simulink model "sampleModel259"  (R2021b)
settings: Solver=VariableStepAuto  StartTime=0.0  StopTime=10.0  RelTol=1e-3
undefined symbols (not defined in the file or in its folder): DiscIntNeverNeededParam
libraries: simulink x9, slpidlib x1
settings Model: Creator=user  LastModifiedBy=user

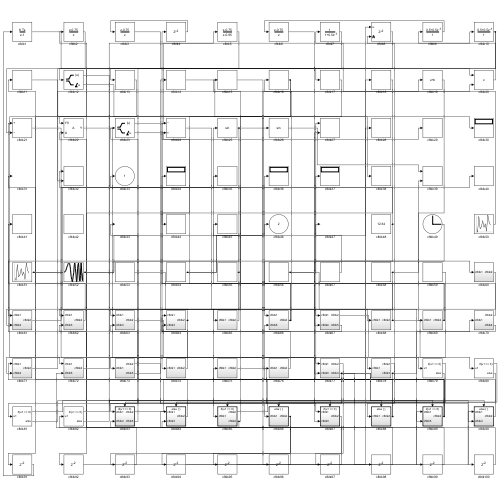
[thumbnail: Simulink's stored preview of the top-level diagram]
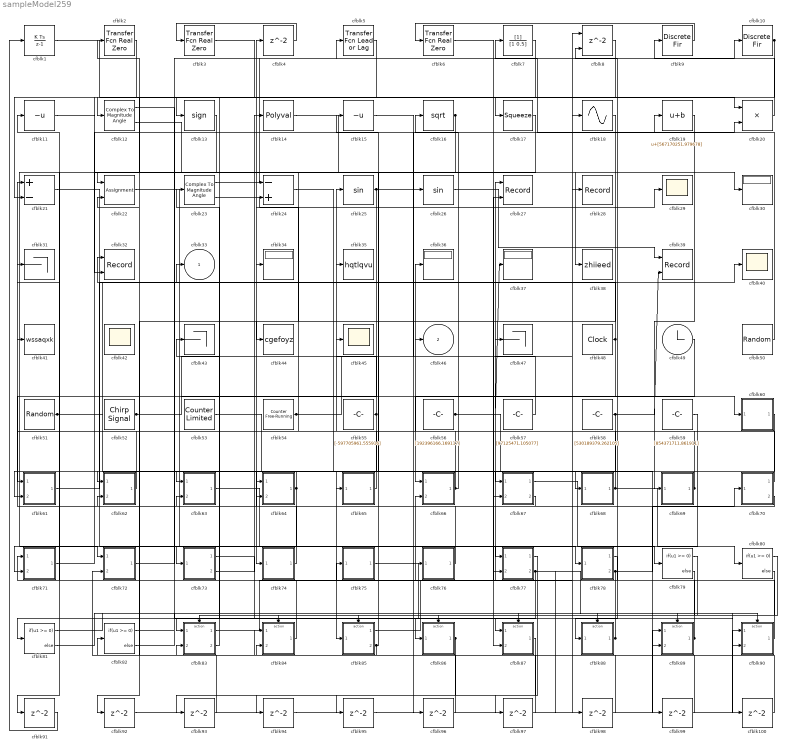
== system sampleModel259 ==
  cfblk1 : DiscreteIntegrator  ICPrevOutput=DiscIntNeverNeededParam  ICPrevScaledInput=DiscIntNeverNeededParam
  cfblk10 : DiscreteFir  SampleTime=1
  cfblk{4,91..100} (11 alike) : Delay  SampleTime=1
  cfblk11 : UnaryMinus
  cfblk12 : ComplexToMagnitudeAngle
  cfblk13 : Signum
  cfblk14 : Polyval  Coefs=[ +2.081618890e-019, -1.441693666e-014, +4.719686976e-010, -8.536869453e-006, +1.621573104e-001, -8.087801117e+001 ]
  cfblk15 : UnaryMinus
  cfblk16 : Sqrt  SaturateOnIntegerOverflow=on
  cfblk17 : Squeeze
  cfblk18 : Sin  TimeSource=Use external signal  SampleTime=0
  cfblk19 : Bias  Bias=[567170251.979678]
  cfblk2 : simulink/Discrete/Transfer Fcn Real Zero  ZeroZ=0.75  ICPrevInput=0.0  DoSatur=off
      settings: SourceProductBaseCode=SL
  cfblk20 : Product  Inputs=**
  cfblk21 : Sum  Inputs=+-
  cfblk22 : Assignment  DiagnosticForDimensions=Warning  IndexOptions=Index vector (dialog)  Indices=1  OutputSizes=1
  cfblk23 : ComplexToMagnitudeAngle
  cfblk24 : Sum  Inputs=-+
  cfblk25 : Trigonometry
  cfblk26 : Trigonometry
  cfblk27 : Record  FileSettingsInternal="{\"entries\":[{\"content\":{\"excelSettings\":{\"content\":{},\"type\":\"Streamout.ExcelSettings\"}},\"type\":\"Streamout.FileSettingStorage\",\"uuid\":\"a15bf5db-3741-4cf3-90f6-61c3119d6459\"}],\"packageUris\":[\"http://schema.mathworks.com/mf0/streamout_blocks/R2020a\"],\"version\":\"1.0\"}"  Layout=[1 1]  SignalsInternal="{\"entries\":[{\"content\":{\"signals\":[{\"content\":{\"blockPath\":[\"sampleModel259/cfblk27\"],\"channel\":[],\"dimensions\":[1],\"domain\":\"sampleModel259/cfblk27\",\"lineColor\":\"#a2142f\",\"plots\":[1],\"port\":1,\"sid\":[\"\"],\"signalID\":10726,\"signalName\":\"cfblk88\"},\"type\":\"RecordBlkView.Signal\",\"uuid\":\"dc7c6215-aa68-4dff-98e1-634e55d8342f\"},{\"content\":{\"blockPath\":[\"sampleModel259/cfblk27\"],\"channel\":[],\"dimensions\":[1],\"domain\":\"sampleModel259/cfblk27\",\"lineColor\":\"#139fff\",\"plots\":[1],\"port\":2,\"sid\":[\"\"],\"signalID\":10730,\"signalName\":\"cfblk85:1\"},\"type\":\"RecordBlkView.Signal\",\"uuid\":\"56125518-63ef-40df-9fd8-c2bea6029bef\"}]},\"type\":\"RecordBlkView.InputSignals\",\"uuid\":\"c2e7fa76-5202-4da8-ac4b-8a415a1de49b\"}],\"packageUris\":[\"http://schema.mathworks.com/mf0/streamout_blocks/R2020a\"],\"version\":\"1.0\"}"  VisualizationBindings="{\"xyplotplugin\":{\"info\":[{\"series\":[{\"bindingParametersList\":[{\"parameter\":\"X-Axis\",\"signalID\":10726,\"signalName\":\"cfblk88\"},{\"parameter\":\"Y-Axis\",\"signalID\":10730,\"signalName\":\"cfblk85:1\"}],\"seriesID\":54620}],\"subplotID\":1}]}}"  CompatibilityTag=XY
  cfblk28 : Record  FileSettingsInternal="{\"entries\":[{\"content\":{\"excelSettings\":{\"content\":{},\"type\":\"Streamout.ExcelSettings\"}},\"type\":\"Streamout.FileSettingStorage\",\"uuid\":\"feed3611-4c3d-457a-aeeb-df4a7c1a2444\"}],\"packageUris\":[\"http://schema.mathworks.com/mf0/streamout_blocks/R2020a\"],\"version\":\"1.0\"}"  SignalsInternal="{\"entries\":[{\"content\":{\"signals\":[{\"content\":{\"blockPath\":[\"sampleModel259/cfblk28\"],\"channel\":[],\"dimensions\":[1],\"domain\":\"sampleModel259/cfblk28\",\"lineColor\":\"#77ac30\",\"plots\":[1],\"port\":1,\"sid\":[\"\"],\"signalID\":10752,\"signalName\":\"cfblk54\"},\"type\":\"RecordBlkView.Signal\",\"uuid\":\"2dff1987-6ee1-4f19-a23b-8245c5550991\"}]},\"type\":\"RecordBlkView.InputSignals\",\"uuid\":\"13ac1fd1-a9dd-4df2-87e5-56531520f03b\"}],\"packageUris\":[\"http://schema.mathworks.com/mf0/streamout_blocks/R2020a\"],\"version\":\"1.0\"}"  VisualizationBindings="{\"sparklinesplugin\":{\"info\":[{\"bindingParametersList\":[],\"subplotID\":1}]}}"
  cfblk{29,40,42,45} (4 alike) : Scope
      cfblk42 settings: Floating=on
  cfblk3 : simulink/Discrete/Transfer Fcn Real Zero  ZeroZ=0.75  ICPrevInput=0.0  DoSatur=off
      settings: SourceProductBaseCode=SL
  cfblk{30,34,36..37} (4 alike) : Display
  cfblk31 : Terminator
  cfblk32 : Record  FileSettingsInternal="{\"entries\":[{\"content\":{\"excelSettings\":{\"content\":{},\"type\":\"Streamout.ExcelSettings\"}},\"type\":\"Streamout.FileSettingStorage\",\"uuid\":\"b89653e3-1f07-4440-8bba-bfd999475c1f\"}],\"packageUris\":[\"http://schema.mathworks.com/mf0/streamout_blocks/R2020a\"],\"version\":\"1.0\"}"  Layout=[1 1]  SignalsInternal="{\"entries\":[{\"content\":{\"signals\":[{\"content\":{\"blockPath\":[\"sampleModel259/cfblk32\"],\"channel\":[],\"dimensions\":[1],\"domain\":\"sampleModel259/cfblk32\",\"lineColor\":\"#a2142f\",\"plots\":[1],\"port\":1,\"sid\":[\"\"],\"signalID\":10734,\"signalName\":\"cfblk48\"},\"type\":\"RecordBlkView.Signal\",\"uuid\":\"aa971696-964b-49ee-93f3-322156b77438\"},{\"content\":{\"blockPath\":[\"sampleModel259/cfblk32\"],\"channel\":[],\"dimensions\":[1],\"domain\":\"sampleModel259/cfblk32\",\"lineColor\":\"#139fff\",\"plots\":[1],\"port\":2,\"sid\":[\"\"],\"signalID\":10738,\"signalName\":\"cfblk7\"},\"type\":\"RecordBlkView.Signal\",\"uuid\":\"a879af8a-cc0a-4d1c-bc44-1debcb7316fc\"}]},\"type\":\"RecordBlkView.InputSignals\",\"uuid\":\"f6f42cd4-c863-4800-b09b-4f72645a5488\"}],\"packageUris\":[\"http://schema.mathworks.com/mf0/streamout_blocks/R2020a\"],\"version\":\"1.0\"}"  VisualizationBindings="{\"xyplotplugin\":{\"info\":[{\"series\":[{\"bindingParametersList\":[{\"parameter\":\"X-Axis\",\"signalID\":10734,\"signalName\":\"cfblk48\"},{\"parameter\":\"Y-Axis\",\"signalID\":10738,\"signalName\":\"cfblk7\"}],\"seriesID\":48673}],\"subplotID\":1}]}}"  CompatibilityTag=XY
  cfblk35 : ToWorkspace  VariableName=hqtlqvu  SaveFormat=Timeseries  SampleTime=-1
  cfblk38 : ToWorkspace  VariableName=zhiieed  SaveFormat=Timeseries  SampleTime=-1
  cfblk39 : Record  FileSettingsInternal="{\"entries\":[{\"content\":{\"excelSettings\":{\"content\":{},\"type\":\"Streamout.ExcelSettings\"}},\"type\":\"Streamout.FileSettingStorage\",\"uuid\":\"77ff0798-a035-4183-a31f-87dc05993ce6\"}],\"packageUris\":[\"http://schema.mathworks.com/mf0/streamout_blocks/R2020a\"],\"version\":\"1.0\"}"  Layout=[1 1]  SignalsInternal="{\"entries\":[{\"content\":{\"signals\":[{\"content\":{\"blockPath\":[\"sampleModel259/cfblk39\"],\"channel\":[],\"dimensions\":[1],\"domain\":\"sampleModel259/cfblk39\",\"lineColor\":\"#a2142f\",\"plots\":[1],\"port\":1,\"sid\":[\"\"],\"signalID\":10742,\"signalName\":\"cfblk26\"},\"type\":\"RecordBlkView.Signal\",\"uuid\":\"7a6bd62a-1676-4e20-b553-acc02f50362f\"},{\"content\":{\"blockPath\":[\"sampleModel259/cfblk39\"],\"channel\":[],\"dimensions\":[1],\"domain\":\"sampleModel259/cfblk39\",\"lineColor\":\"#139fff\",\"plots\":[1],\"port\":2,\"sid\":[\"\"],\"signalID\":10746,\"signalName\":\"cfblk58\"},\"type\":\"RecordBlkView.Signal\",\"uuid\":\"c6f9d57b-6e52-40c4-aa5d-954adbceaf7c\"}]},\"type\":\"RecordBlkView.InputSignals\",\"uuid\":\"08c0dad2-ea46-41f9-9f49-8bf2c65fcba6\"}],\"packageUris\":[\"http://schema.mathworks.com/mf0/streamout_blocks/R2020a\"],\"version\":\"1.0\"}"  VisualizationBindings="{\"xyplotplugin\":{\"info\":[{\"series\":[{\"bindingParametersList\":[{\"parameter\":\"X-Axis\",\"signalID\":10742,\"signalName\":\"cfblk26\"},{\"parameter\":\"Y-Axis\",\"signalID\":10746,\"signalName\":\"cfblk58\"}],\"seriesID\":17387}],\"subplotID\":1}]}}"  CompatibilityTag=XY
  cfblk41 : ToWorkspace  VariableName=wssaqxk  SaveFormat=Timeseries  SampleTime=-1
  cfblk43 : Terminator
  cfblk44 : ToWorkspace  VariableName=cgefoyz  SaveFormat=Timeseries  SampleTime=-1
  cfblk47 : Terminator
  cfblk48 : DigitalClock
  cfblk49 : Clock
  cfblk5 : simulink/Discrete/Transfer Fcn Lead or Lag  PoleZ=0.95  ZeroZ=0.75  ICPrevOutput=0.0  ICPrevInput=0.0  DoSatur=off
      settings: SourceProductBaseCode=SL
  cfblk50 : UniformRandomNumber  Minimum=[-9722096741.115524]  Maximum=[1390579412.419839]  Seed=[42070963.000000]  SampleTime=0.1
  cfblk51 : UniformRandomNumber  Minimum=[-9203084718.990440]  Maximum=[862788359.237772]  Seed=[70444919.000000]  SampleTime=0.1
  cfblk52 : simulink/Sources/Chirp Signal  f1=[435243080.422946]  T=[-898675247.120683]  f2=[958327382.414222]
  cfblk53 : simulink/Sources/Counter Limited  uplimit=[732.000000]  tsamp=-1
  cfblk54 : simulink/Sources/Counter Free-Running  NumBits=[39.000000]  tsamp=-1
  cfblk55 : Constant  Value=[-597705961.555916]  SampleTime=1
  cfblk56 : Constant  Value=[192396166.169117]  SampleTime=1
  cfblk57 : Constant  Value=[97125471.105077]  SampleTime=1
  cfblk58 : Constant  Value=[530189379.262105]  SampleTime=1
  cfblk59 : Constant  Value=[854371711.861911]  SampleTime=1
  cfblk6 : simulink/Discrete/Transfer Fcn Real Zero  ZeroZ=0.75  ICPrevInput=0.0  DoSatur=off
      settings: SourceProductBaseCode=SL
  cfblk60 : Subsystem
  cfblk61 : Subsystem
  cfblk62 : Subsystem
  cfblk63 : Subsystem
  cfblk64 : Subsystem
  cfblk65 : Subsystem
  cfblk66 : Subsystem
  cfblk67 : Subsystem
  cfblk68 : Subsystem
  cfblk69 : Subsystem
  cfblk7 : DiscreteFilter  SampleTime=1
  cfblk70 : Subsystem
  cfblk71 : Subsystem
  cfblk72 : Subsystem
  cfblk73 : Subsystem
  cfblk74 : Subsystem
  cfblk75 : Subsystem
  cfblk76 : Subsystem
  cfblk77 : Subsystem
  cfblk78 : Subsystem
  cfblk{79..82} (4 alike) : If  IfExpression=u1 >= 0  SampleTime=1
  cfblk8 : Delay  ShowEnablePort=on  SampleTime=1
      settings: InputPortMap=u0,e6
  cfblk83 : Subsystem  TreatAsAtomicUnit=on
  cfblk84 : Subsystem  TreatAsAtomicUnit=on
  cfblk85 : Subsystem  TreatAsAtomicUnit=on
  cfblk86 : Subsystem  TreatAsAtomicUnit=on
  cfblk87 : Subsystem  TreatAsAtomicUnit=on
  cfblk88 : Subsystem  TreatAsAtomicUnit=on
  cfblk89 : Subsystem  TreatAsAtomicUnit=on
  cfblk9 : DiscreteFir  SampleTime=1
  cfblk90 : Subsystem  TreatAsAtomicUnit=on
  cfblk33 : Outport
  cfblk46 : Outport  Port=2
  wires:
  cfblk69/1(cfblk2) -> cfblk25/1, cfblk15/1
  cfblk61/1(cfblk2) -> cfblk35/1
  cfblk59/1 -> cfblk73/1(cfblk1)
  cfblk26/1 -> cfblk39/1
  cfblk17/1 -> cfblk72/1(cfblk1)
  cfblk88/1(cfblk2) -> cfblk27/1, cfblk31/1
  cfblk2/1 -> cfblk12/1
  cfblk68/1(cfblk2) -> cfblk80/1, cfblk34/1
  cfblk67/1(cfblk2) -> cfblk79/1
  cfblk20/1 -> cfblk9/1
  cfblk9/1 -> cfblk6/1
  cfblk22/1 -> cfblk78/1(cfblk1)
  cfblk74/1(cfblk2) -> cfblk4/1
  cfblk21/1 -> cfblk77/1(cfblk1)
  cfblk54/1 -> cfblk36/1, cfblk28/1
  cfblk60/1(cfblk2) -> cfblk74/1(cfblk1)
  cfblk4/1 -> cfblk3/1
  cfblk53/1 -> cfblk85/1(cfblk1)
  cfblk85/1(cfblk2) -> cfblk27/2
  cfblk8/1 -> cfblk22/1
  cfblk75/1(cfblk2) -> cfblk87/1(cfblk1)
  cfblk49/1 -> cfblk66/1(cfblk1)
  cfblk58/1 -> cfblk39/2, cfblk61/2(cfblk4)
  cfblk65/1(cfblk2) -> cfblk21/1
  cfblk63/1(cfblk2) -> cfblk87/2(cfblk3)
  cfblk14/1 -> cfblk38/1
  cfblk56/1 -> cfblk37/1, cfblk89/2(cfblk5)
  cfblk3/1 -> cfblk20/1
  cfblk57/1 -> cfblk47/1
  cfblk51/1 -> cfblk77/2(cfblk3), cfblk40/1
  cfblk23/1 -> cfblk10/1
  cfblk84/1(cfblk2) -> cfblk43/1
  cfblk71/1(cfblk2) -> cfblk19/1
  cfblk16/1 -> cfblk65/1(cfblk1), cfblk44/1
  cfblk67/2(cfblk5) -> cfblk64/1(cfblk1)
  cfblk1/1 -> cfblk17/1
  cfblk76/1(cfblk2) -> cfblk41/1
  cfblk89/1(cfblk2) -> cfblk75/1(cfblk1), cfblk63/2(cfblk3), cfblk62/2(cfblk3), cfblk8/2
  cfblk19/1 -> cfblk69/1(cfblk1)
  cfblk48/1 -> cfblk32/1, cfblk67/2(cfblk4)
  cfblk73/1(cfblk2) -> cfblk86/1(cfblk1)
  cfblk64/1(cfblk2) -> cfblk62/1(cfblk1), cfblk71/2(cfblk4)
  cfblk50/1 -> cfblk7/1
  cfblk73/2(cfblk3) -> cfblk14/1
  cfblk72/1(cfblk2) -> cfblk5/1
  cfblk5/1 -> cfblk13/1
  cfblk23/2 -> cfblk29/1
  cfblk6/1 -> cfblk68/1(cfblk1)
  cfblk11/1 -> cfblk30/1
  cfblk85/2(cfblk4) -> cfblk72/2(cfblk5), cfblk33/1
  cfblk12/1 -> cfblk90/2(cfblk4)
  cfblk52/1 -> cfblk26/1, cfblk60/1(cfblk1)
  cfblk86/1(cfblk2) -> cfblk94/1, cfblk95/1
  cfblk90/1(cfblk2) -> cfblk66/2(cfblk5)
  cfblk70/1(cfblk2) -> cfblk46/1
  cfblk77/2(cfblk4) -> cfblk81/1, cfblk98/1, cfblk99/1, cfblk100/1
  cfblk78/1(cfblk2) -> cfblk88/1(cfblk1)
  cfblk78/2(cfblk3) -> cfblk71/1(cfblk1), cfblk70/1(cfblk1)
  cfblk12/2 -> cfblk76/1(cfblk1)
  cfblk70/2(cfblk4) -> cfblk64/2(cfblk3)
  cfblk62/1(cfblk2) -> cfblk11/1
  cfblk83/1(cfblk2) -> cfblk18/1
  cfblk25/1 -> cfblk20/2, cfblk61/1(cfblk1)
  cfblk55/1 -> cfblk83/1(cfblk1), cfblk45/1
  cfblk7/1 -> cfblk32/2
  cfblk10/1 -> cfblk21/2, cfblk63/1(cfblk1)
  cfblk66/1(cfblk2) -> cfblk24/1, cfblk16/1, cfblk24/2
  cfblk83/2(cfblk5) -> cfblk23/1
  cfblk24/1 -> cfblk67/1(cfblk1)
  cfblk79/1 -> cfblk83/Action
  cfblk79/2 -> cfblk84/Action
  cfblk80/1 -> cfblk85/Action
  cfblk80/2 -> cfblk86/Action
  cfblk81/1 -> cfblk87/Action
  cfblk81/2 -> cfblk88/Action
  cfblk82/1 -> cfblk89/Action
  cfblk82/2 -> cfblk90/Action
  cfblk13/1 -> cfblk91/1
  cfblk91/1 -> cfblk1/1
  cfblk18/1 -> cfblk92/1
  cfblk92/1 -> cfblk90/1(cfblk1)
  cfblk87/1(cfblk2) -> cfblk93/1
  cfblk93/1 -> cfblk2/1
  cfblk94/1 -> cfblk89/1(cfblk1)
  cfblk95/1 -> cfblk8/1
  cfblk15/1 -> cfblk96/1
  cfblk96/1 -> cfblk22/2
  cfblk77/1(cfblk2) -> cfblk97/1
  cfblk97/1 -> cfblk82/1
  cfblk98/1 -> cfblk83/2(cfblk4)
  cfblk99/1 -> cfblk84/1(cfblk1)
  cfblk100/1 -> cfblk84/2(cfblk3)

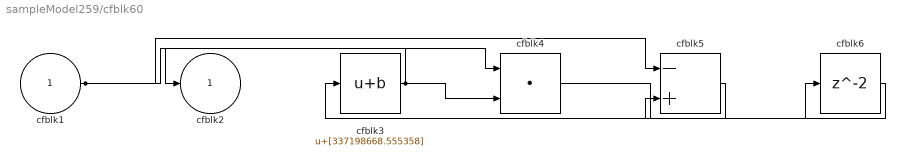
== system sampleModel259/cfblk60 ==
  cfblk1 : Inport
  cfblk3 : Bias  Bias=[337198668.555358]
  cfblk4 : DotProduct  InputSameDT=on  OutDataTypeStr=Inherit: Inherit via internal rule
  cfblk5 : Sum  Inputs=-+
  cfblk6 : Delay  SampleTime=1
  cfblk2 : Outport
  wires:
  cfblk3/1 -> cfblk2/1, cfblk4/2
  cfblk1/1 -> cfblk5/1, cfblk4/1
  cfblk5/1 -> cfblk3/1
  cfblk4/1 -> cfblk6/1
  cfblk6/1 -> cfblk5/2

== system sampleModel259/cfblk61 ==
  cfblk1 : Inport
  cfblk4 : Inport  Port=2
  cfblk3 : Product  Inputs=**
  cfblk2 : Outport
  wires:
  cfblk1/1 -> cfblk2/1, cfblk3/2
  cfblk4/1 -> cfblk3/1

== system sampleModel259/cfblk62 ==
  cfblk1 : Inport
  cfblk3 : Inport  Port=2
  cfblk2 : Outport
  wires:
  cfblk3/1 -> cfblk2/1

== system sampleModel259/cfblk63 ==
  cfblk1 : Inport
  cfblk3 : Inport  Port=2
  cfblk2 : Outport
  wires:
  cfblk1/1 -> cfblk2/1

== system sampleModel259/cfblk64 ==
  cfblk1 : Inport
  cfblk3 : Inport  Port=2
  cfblk2 : Outport
  wires:
  cfblk1/1 -> cfblk2/1

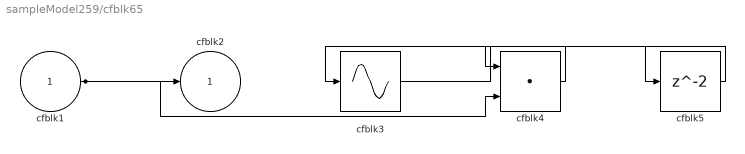
== system sampleModel259/cfblk65 ==
  cfblk1 : Inport
  cfblk3 : Sin  TimeSource=Use external signal  SampleTime=0
  cfblk4 : DotProduct  InputSameDT=on  OutDataTypeStr=Inherit: Inherit via internal rule
  cfblk5 : Delay  SampleTime=1
  cfblk2 : Outport
  wires:
  cfblk1/1 -> cfblk2/1, cfblk4/2
  cfblk4/1 -> cfblk3/1
  cfblk3/1 -> cfblk5/1
  cfblk5/1 -> cfblk4/1

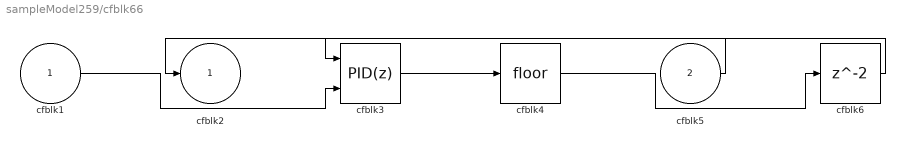
== system sampleModel259/cfblk66 ==
  cfblk1 : Inport
  cfblk5 : Inport  Port=2
  cfblk3 : slpidlib/PID Controller (2DOF)  Controller=PID  Form=Parallel  TimeDomain=Discrete-time  UseExternalTs=off  SampleTime=1  IntegratorMethod=Forward Euler  FilterMethod=Forward Euler  ControllerParametersSource=internal  P=1  I=1  D=0  UseFilter=on  N=100  b=1  c=1  TunerSelectOption=Transfer Function Based (PID Tuner App)  InitialConditionSource=internal  InitialConditionForIntegrator=0  InitialConditionForFilter=0  DifferentiatorICPrevScaledInput=0  ExternalReset=none  TrackingMode=off  Kt=1  LimitOutput=off  SatLimitsSource=internal  UpperSaturationLimit=inf  LowerSaturationLimit=-inf  LinearizeAsGain=off  AntiWindupMode=none  Kb=1  POutMin=[]  POutMax=[]  IOutMin=[]  IOutMax=[]  DOutMin=[]  DOutMax=[]  NOutMin=[]  NOutMax=[]  bOutMin=[]  bOutMax=[]  cOutMin=[]  cOutMax=[]  SumOutMin=[]  SumOutMax=[]  SaturationOutMin=[]  SaturationOutMax=[]  PParamMin=[]  PParamMax=[]  IParamMin=[]  IParamMax=[]  DParamMin=[]  DParamMax=[]  NParamMin=[]  NParamMax=[]  bParamMin=[]  bParamMax=[]  cParamMin=[]  cParamMax=[]  KbParamMin=[]  KbParamMax=[]  KtParamMin=[]  KtParamMax=[]  KbOutMin=[]  KbOutMax=[]  KtOutMin=[]  KtOutMax=[]  IntegratorOutMin=[]  IntegratorOutMax=[]  FilterOutMin=[]  FilterOutMax=[]  SumI1OutMin=[]  SumI1OutMax=[]  SumI2OutMin=[]  SumI2OutMax=[]  SumI3OutMin=[]  SumI3OutMax=[]  SumI4OutMin=[]  SumI4OutMax=[]  SumDOutMin=[]  SumDOutMax=[]  Sum1OutMin=[]  Sum1OutMax=[]  Sum2OutMin=[]  Sum2OutMax=[]  Sum3OutMin=[]  Sum3OutMax=[]  DifferentiatorOutMin=[]  DifferentiatorOutMax=[]  FilterDiffOutCoefMin=[]  FilterDiffOutCoefMax=[]  ReciprocalOutMin=[]  ReciprocalOutMax=[]  SumDenOutMin=[]  SumDenOutMax=[]  SumNumOutMin=[]  SumNumOutMax=[]  DivideOutMin=[]  DivideOutMax=[]  UdiffTsProdOutMin=[]  UdiffTsProdOutMax=[]  NTsProdOutMin=[]  NTsProdOutMax=[]  UintegralTsProdOutMin=[]  UintegralTsProdOutMax=[]  UngainTsProdOutMin=[]  UngainTsProdOutMax=[]  IntegratorContinuousStateAttributes=''  IntegratorStateMustResolveToSignalObject=off  IntegratorRTWStateStorageClass=Auto  FilterContinuousStateAttributes=''  FilterStateMustResolveToSignalObject=off  FilterRTWStateStorageClass=Auto  ParallelPVariant=InternalParameters  IdealPVariant=Disabled  IVariant=InternalParameters  DVariant=InternalParameters  bVariant=InternalParameters  cVariant=InternalParameters  IntegratorVariant=Discrete  SatVariant=Disabled  AWVariant=Passthrough  PCopyVariant=Disabled  TRVariant=Disabled  FdbkBlocksVariant=Forward  IdealPFdbkVariant=Disabled  SatFdbkVariant=Disabled  DerivativeFilterVariant=ForwardEulerFilter  NVariant=InternalParameters  NCopyVariant=Disabled  FilterICVariant=InternalICsFilter  IntegratorICVariant=InternalICs  ExternalResetVariant=Disabled  TRSumVariant=Passthrough  SumFdbkVariant=Disabled  SumVariant=Sum_PID  TsampFilterVariant=InternalTs  TsampNgainVariant=Passthrough  TsampIntegralVariant=Passthrough  ExternalSaturationOutDataTypeStr=Inherit: Same as second input
      settings: SourceProductBaseCode=SL
  cfblk4 : Rounding
  cfblk6 : Delay  SampleTime=1
  cfblk2 : Outport
  wires:
  cfblk3/1 -> cfblk4/1
  cfblk5/1 -> cfblk2/1
  cfblk1/1 -> cfblk3/2
  cfblk4/1 -> cfblk6/1
  cfblk6/1 -> cfblk3/1

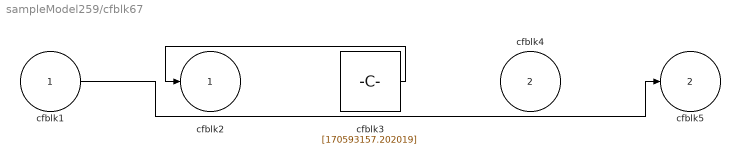
== system sampleModel259/cfblk67 ==
  cfblk1 : Inport
  cfblk4 : Inport  Port=2
  cfblk3 : Constant  Value=[170593157.202019]  SampleTime=1
  cfblk2 : Outport
  cfblk5 : Outport  Port=2
  wires:
  cfblk3/1 -> cfblk2/1
  cfblk1/1 -> cfblk5/1

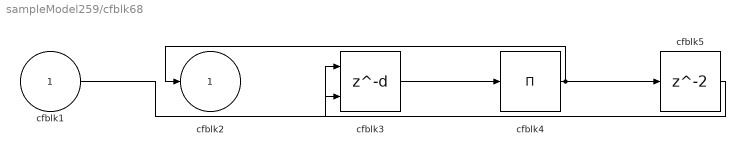
== system sampleModel259/cfblk68 ==
  cfblk1 : Inport
  cfblk3 : Delay  DelayLengthSource=Input port  SampleTime=1
      settings: InputPortMap=u0,p1
  cfblk4 : Product  Inputs=*
  cfblk5 : Delay  SampleTime=1
  cfblk2 : Outport
  wires:
  cfblk4/1 -> cfblk2/1, cfblk5/1
  cfblk3/1 -> cfblk4/1
  cfblk1/1 -> cfblk3/1
  cfblk5/1 -> cfblk3/2

== system sampleModel259/cfblk69 ==
  cfblk1 : Inport
  cfblk3 : simulink/Discrete/Tapped Delay  vinit=0.0  samptime=-1  NumDelays=1  DelayOrder=Oldest  includeCurrent=off
  cfblk4 : Sqrt  SaturateOnIntegerOverflow=on
  cfblk2 : Outport
  wires:
  cfblk1/1 -> cfblk3/1
  cfblk3/1 -> cfblk2/1, cfblk4/1

== system sampleModel259/cfblk70 ==
  cfblk1 : Inport
  cfblk3 : Constant  Value=[-642189486.966722]  SampleTime=1
  cfblk2 : Outport
  cfblk4 : Outport  Port=2
  wires:
  cfblk3/1 -> cfblk4/1
  cfblk1/1 -> cfblk2/1

== system sampleModel259/cfblk71 ==
  cfblk1 : Inport
  cfblk4 : Inport  Port=2
  cfblk3 : simulink/Discrete/Difference  ICPrevInput=0.0  OutMin=[]  OutMax=[]  OutDataTypeStr=Inherit: Inherit via back propagation  OutDataType=fixdt(1, 16)  OutScaling=2^-10  DoSatur=off
  cfblk2 : Outport
  wires:
  cfblk3/1 -> cfblk2/1
  cfblk4/1 -> cfblk3/1

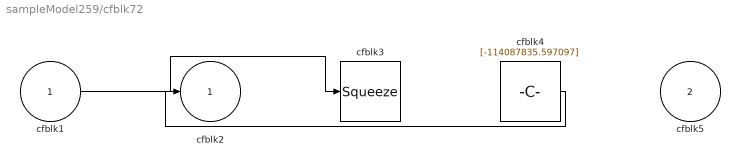
== system sampleModel259/cfblk72 ==
  cfblk1 : Inport
  cfblk5 : Inport  Port=2
  cfblk3 : Squeeze
  cfblk4 : Constant  Value=[-114087835.597097]  SampleTime=1
  cfblk2 : Outport
  wires:
  cfblk1/1 -> cfblk3/1
  cfblk4/1 -> cfblk2/1

== system sampleModel259/cfblk73 ==
  cfblk1 : Inport
  cfblk2 : Outport
  cfblk3 : Outport  Port=2
  wires:
  cfblk1/1 -> cfblk2/1, cfblk3/1

== system sampleModel259/cfblk74 ==
  cfblk1 : Inport
  cfblk3 : DiscreteFir  SampleTime=1
  cfblk2 : Outport
  wires:
  cfblk1/1 -> cfblk3/1
  cfblk3/1 -> cfblk2/1

== system sampleModel259/cfblk75 ==
  cfblk1 : Inport
  cfblk3 : UnaryMinus
  cfblk2 : Outport
  wires:
  cfblk1/1 -> cfblk3/1
  cfblk3/1 -> cfblk2/1

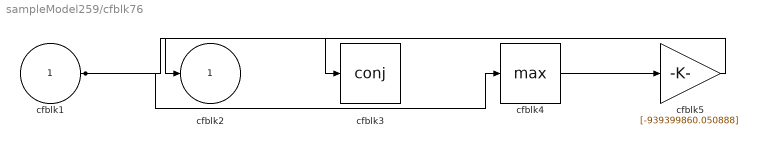
== system sampleModel259/cfblk76 ==
  cfblk1 : Inport
  cfblk3 : Math  Operator=conj  SaturateOnIntegerOverflow=on
  cfblk4 : MinMax  Function=max
  cfblk5 : Gain  Gain=[-939399860.050888]
  cfblk2 : Outport
  wires:
  cfblk4/1 -> cfblk5/1
  cfblk5/1 -> cfblk2/1
  cfblk1/1 -> cfblk4/1, cfblk3/1

== system sampleModel259/cfblk77 ==
  cfblk1 : Inport
  cfblk3 : Inport  Port=2
  cfblk2 : Outport
  cfblk4 : Outport  Port=2
  wires:
  cfblk3/1 -> cfblk4/1
  cfblk1/1 -> cfblk2/1

== system sampleModel259/cfblk78 ==
  cfblk1 : Inport
  cfblk2 : Outport
  cfblk3 : Outport  Port=2
  wires:
  cfblk1/1 -> cfblk2/1, cfblk3/1

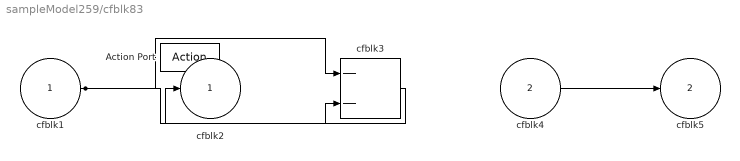
== system sampleModel259/cfblk83 ==
  cfblk1 : Inport
  cfblk4 : Inport  Port=2
  Action Port : ActionPort  ActionPortLabel=if(u1 >= 0)
  cfblk3 : Sum  Inputs=--
  cfblk2 : Outport
  cfblk5 : Outport  Port=2
  wires:
  cfblk4/1 -> cfblk5/1
  cfblk3/1 -> cfblk2/1
  cfblk1/1 -> cfblk3/1, cfblk3/2

== system sampleModel259/cfblk84 ==
  cfblk1 : Inport
  cfblk3 : Inport  Port=2
  Action Port : ActionPort  ActionPortLabel=else
  cfblk2 : Outport
  wires:
  cfblk3/1 -> cfblk2/1

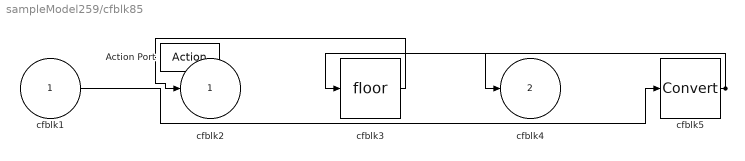
== system sampleModel259/cfblk85 ==
  cfblk1 : Inport
  Action Port : ActionPort  ActionPortLabel=if(u1 >= 0)
  cfblk3 : Rounding
  cfblk5 : DataTypeConversion
  cfblk2 : Outport
  cfblk4 : Outport  Port=2
  wires:
  cfblk1/1 -> cfblk5/1
  cfblk3/1 -> cfblk2/1
  cfblk5/1 -> cfblk3/1, cfblk4/1

== system sampleModel259/cfblk86 ==
  cfblk1 : Inport
  Action Port : ActionPort  ActionPortLabel=else
  cfblk3 : Constant  Value=[-329889022.897536]  SampleTime=1
  cfblk2 : Outport
  wires:
  cfblk1/1 -> cfblk2/1

== system sampleModel259/cfblk87 ==
  cfblk1 : Inport
  cfblk3 : Inport  Port=2
  Action Port : ActionPort  ActionPortLabel=if(u1 >= 0)
  cfblk2 : Outport
  wires:
  cfblk1/1 -> cfblk2/1

== system sampleModel259/cfblk88 ==
  cfblk1 : Inport
  Action Port : ActionPort  ActionPortLabel=else
  cfblk3 : DiscreteFilter
  cfblk2 : Outport
  wires:
  cfblk1/1 -> cfblk2/1, cfblk3/1

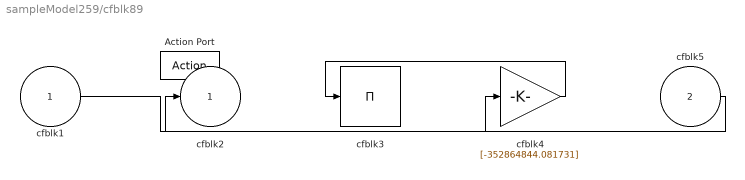
== system sampleModel259/cfblk89 ==
  cfblk1 : Inport
  cfblk5 : Inport  Port=2
  Action Port : ActionPort  ActionPortLabel=if(u1 >= 0)
  cfblk3 : Product  Inputs=*
  cfblk4 : Gain  Gain=[-352864844.081731]
  cfblk2 : Outport
  wires:
  cfblk4/1 -> cfblk3/1
  cfblk5/1 -> cfblk2/1
  cfblk1/1 -> cfblk4/1

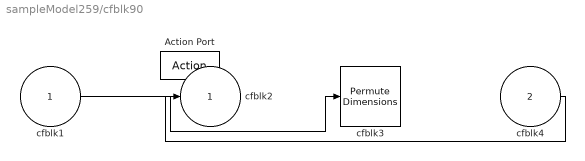
== system sampleModel259/cfblk90 ==
  cfblk1 : Inport
  cfblk4 : Inport  Port=2
  Action Port : ActionPort  ActionPortLabel=else
  cfblk3 : PermuteDimensions
  cfblk2 : Outport
  wires:
  cfblk1/1 -> cfblk3/1
  cfblk4/1 -> cfblk2/1
